simulink model "polymultgf2_test"  (R2020b)
settings: Solver=FixedStepAuto  StartTime=0.0  StopTime=10.0  RelTol=1e-3  EnableMultiTasking=on
settings Model: SILPILModeSetting=veronly  ExtModeTrigDuration=2  Creator=Dona  LastModifiedBy=tcbir
settings OptimizationCC: EnhancedBackFolding=on  PassReuseOutputArgsAs=Individual arguments  ZeroExternalMemoryAtStartup=off  ZeroInternalMemoryAtStartup=off  MaxStackSize=64  OptimizeBlockOrder=speed  DifferentSizesBufferReuse=on  OptimizationCustomize=off  EfficientTunableParamExpr=on
settings DebuggingCC: ParameterTunabilityLossMsg=error
settings HardwareCC: ProdBitPerInt=16  ProdBitPerPointer=16  ProdBitPerSizeT=16  ProdBitPerPtrDiffT=16  ProdLargestAtomicFloat=None  ProdWordSize=8  ProdHWDeviceType=Atmel->AVR  UseEmbeddedCoderFeatures=off  UseSimulinkCoderFeatures=off
settings SFSimCC: MATLABDynamicMemAlloc=off
settings RTWCC: Description=Embedded Coder  SystemTargetFile=ert.tlc  HardwareBoard=Arduino Mega 2560  TemplateMakefile=ert_default_tmf  Toolchain=Arduino AVR  BuildConfiguration=Faster Runs
settings CodeAppCC: ForceParamTrailComments=on  IgnoreCustomStorageClasses=off  OperatorAnnotations=on  SimulinkDataObjDesc=on  SFDataObjDesc=on  InsertBlockDesc=on
settings ERTTargetCC: SupportContinuousTime=on  SupportNonInlinedSFcns=on  SupportVariableSizeSignals=on  ExtModeStaticAllocSize=2048

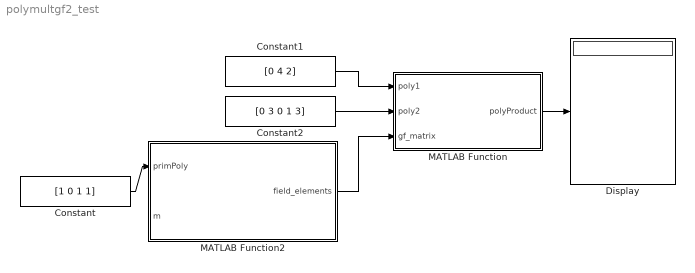
== system polymultgf2_test ==
  Constant : Constant  Value=[1 0 1 1]
  Constant1 : Constant  Value=[0 4 2]  VectorParams1D=off
  Constant2 : Constant  Value=[0 3 0 1 3]  VectorParams1D=off
  Display : Display
  MATLAB Function : MATLAB Function  TreatAsAtomicUnit=on
  MATLAB Function2 : MATLAB Function  TreatAsAtomicUnit=on
  wires:
  Constant/1 -> MATLAB Function2/1(primPoly)
  MATLAB Function2/1(field_elements) -> MATLAB Function/3(gf_matrix)
  Constant2/1 -> MATLAB Function/2(poly2)
  Constant1/1 -> MATLAB Function/1(poly1)
  MATLAB Function/1(polyProduct) -> Display/1

== matlab function polymultgf2_test/MATLAB Function2 ==
  data: primPoly input; field_elements output; m input
% GenerateGF2m: generates the selected Galois Field element. The inputs should be the
% order m and the coefficients of an appropriate primitive polynomial. The generated field,
% in either binary or power notation, may be a calling parameter for each of the other
% functions. Hint: I strongly suggest that you input the coefficients in “power” notation,
% with the highest order power on the left

function field_elements  = GenerateGF2m(primPoly, m) %primPoly in power notation, highest order on left

m = 3;
% hard coded size of retrun matrices and gf mtrix because simulink
% whines about variable output size. Havent figured out how to fix it
% ask laberge
gf = zeros(8, 3); %there are 2^m field elements
field_elements = zeros(8, 3); %there are 2^m field elements

gfIndx = 2; %gfIndx(1) holds initial state 
numShifts = (2^m) - 1;
s_reg = zeros(1,int8(m));
s_reg(end) = 1; %rightmost element of init shr is 1
gf(1, :) = 0;%write the contents of the init shift register to the matrix of gf elements
gf(2, :) = s_reg;
for i = 2:numShifts %number of shifts corresponds to power of primitive element
    carryOut = s_reg(1);%save the value to be wrapped
    for i0 = 1:numel(s_reg)-1
        if primPoly(i0 + 1) == 1
            s_reg(i0) = xor(carryOut, s_reg(i0 + 1));
        else
            s_reg(i0) = s_reg(i0 + 1);
        end
    end
    s_reg(end) = carryOut;
    gf(i+1,:) = s_reg; %add the newly shifted register to the gf matrix
end
field_elements = gf;
end

== matlab function polymultgf2_test/MATLAB Function ==
  data: poly1 input; poly2 input; gf_matrix input; polyProduct output
% Multiply two polynomials over GF(2m)[x] , with arithmetic in that field.
% I expect that this function will use the previous functions, as necessary. Hint 1: I suggest
% using power notation for the calling parameters and the returned parameter. Hint 2: this
% will essentially do a convolution with arithmetic in the Big Field. The MATLAB routine
% conv will not do the correct algebra and so should not be used!
function polyProduct  = PolyMultGF2m(poly1, poly2, gf_matrix)
m = numel(gf_matrix(1,:));
offset = 0; 
rowIndx = 1;
power1 = numel(poly1)-1;% deg(poly1)
power2 = numel(poly2)-1;% deg(poly2)
colIndx = power1+power2+1;
toAdd = -1*ones(power2+1,colIndx); % (# elements poly2, total # elements)


for i = numel(poly2): -1: 1 %for each part of poly2 from right to left
    for j = numel(poly1(1,:)): -1: 1 %for each element of poly 1 from right to left
        
        % do we need the multGFM function if i can just check if either of
        % them are inf
        p = MultGF2m(poly2(i),poly1(j), gf_matrix);%multiply each element of poly1 by the poly2 element
        if(p < 0)
            toAdd(rowIndx, colIndx - offset) = -1;
        else
            toAdd(rowIndx, colIndx - offset) = p;
        end
        colIndx = colIndx - 1;%go to next column (move left)
    end
    offset = offset + 1; %increment offset and row
    rowIndx = rowIndx + 1;
    colIndx = power1+power2+1; %reset column index to rightmost place
end
 
sum = -1*ones(1,power1+power2+1);
%add the rows from multiplication
[row, col] = size(toAdd);
sum(1,:) = toAdd(1, :);
for i0 = 2:(row) %for each row after the first
    for i1 = numel(sum):-1:1 %for each row element right to left
        in1 = toAdd(i0, i1);
        in2 = sum(1, i1);
        sum(1,i1) = AddGF2m(in1, in2, gf_matrix);%add that element and the corresponding first row element
    end
end
polyProduct = sum;
end
